simulink model "sfunction"  (R2022b)
settings: Solver=VariableStepAuto  StartTime=0.0  StopTime=2  RelTol=1e-3
libraries: fuzblock x2
settings Model: Creator=ericliu  LastModifiedBy=Lenovo
settings OptimizationCC: ReuseModelBlockBuffer=on
settings RTWCC: GPUComputeCapability=5.0

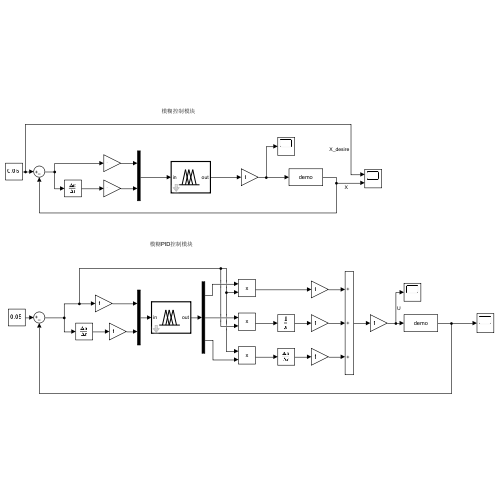
[thumbnail: Simulink's stored preview of the top-level diagram]
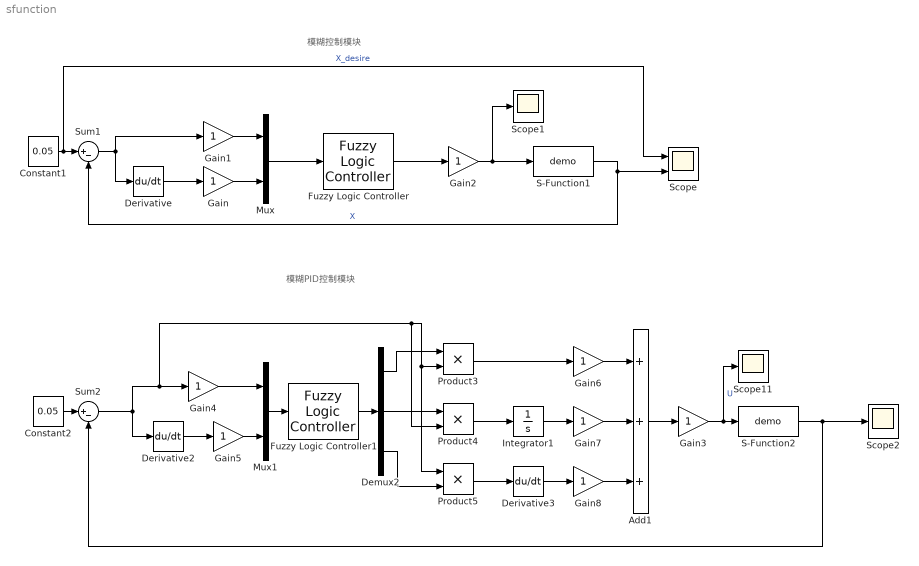
== system sfunction ==
  note: 模糊控制模块
  note: 模糊PID控制模块
  Add1 : Sum  Inputs=+++
  Constant1 : Constant  Value=0.05
  Constant2 : Constant  Value=0.05
  Demux2 : Demux  Outputs=3
  Derivative : Derivative
  Derivative2 : Derivative
  Derivative3 : Derivative
  Fuzzy Logic Controller : fuzblock/Fuzzy Logic  Controller  FIS='fuzzy1.fis'  OutputSampleNumber=101  DataType=double  FuzzifiedInputs=off  RuleFiringStrengths=off  RuleOutputs=off  AggregatedOutputs=off  SimulateUsing=Interpreted execution  OutOfRangeInputValueMessage=warning  NoRuleFiredMessage=warning  EmptyOutputFuzzySetMessage=warning
  Fuzzy Logic Controller1 : fuzblock/Fuzzy Logic  Controller  FIS='PIDfuzzy1.fis'  OutputSampleNumber=101  DataType=double  FuzzifiedInputs=off  RuleFiringStrengths=off  RuleOutputs=off  AggregatedOutputs=off  SimulateUsing=Interpreted execution  OutOfRangeInputValueMessage=warning  NoRuleFiredMessage=warning  EmptyOutputFuzzySetMessage=warning
  Gain{,1..8} (9 alike) : Gain
  Integrator1 : Integrator
  Mux : Mux  Inputs=2
  Mux1 : Mux  Inputs=2
  Product3 : Product
  Product4 : Product
  Product5 : Product
  S-Function1 : S-Function  FunctionName=demo  SFunctionDeploymentMode=off  EnableBusSupport=off
  S-Function2 : S-Function  FunctionName=demo  SFunctionDeploymentMode=off  EnableBusSupport=off
  Scope : Scope  NumInputPorts=2
  Scope1 : Scope
  Scope11 : Scope
  Scope2 : Scope
  Sum1 : Sum  Inputs=|+-
  Sum2 : Sum  Inputs=|+-
  wires:
  Mux/1 -> Fuzzy Logic Controller/1
  S-Function1/1 -> Scope/2, Sum1/2  "X"
  Sum1/1 -> Derivative/1, Gain1/1
  Gain1/1 -> Mux/1
  Derivative/1 -> Gain/1
  Gain/1 -> Mux/2
  Fuzzy Logic Controller/1 -> Gain2/1
  Gain2/1 -> Scope1/1, S-Function1/1
  Constant1/1 -> Scope/1, Sum1/1  "X_desire"
  Product4/1 -> Integrator1/1
  Fuzzy Logic Controller1/1 -> Demux2/1
  Gain4/1 -> Mux1/1
  Derivative2/1 -> Gain5/1
  Mux1/1 -> Fuzzy Logic Controller1/1
  Demux2/1 -> Product3/1
  Product5/1 -> Derivative3/1
  Add1/1 -> Gain3/1
  Integrator1/1 -> Gain7/1
  Gain8/1 -> Add1/3
  Product3/1 -> Gain6/1
  Gain7/1 -> Add1/2
  Derivative3/1 -> Gain8/1
  Gain3/1 -> Scope11/1, S-Function2/1  "U"
  Demux2/2 -> Product4/1
  Gain5/1 -> Mux1/2
  Demux2/3 -> Product5/2
  Gain6/1 -> Add1/1
  Sum2/1 -> Derivative2/1, Product5/1, Product3/2, Product4/2, Gain4/1
  Constant2/1 -> Sum2/1
  S-Function2/1 -> Scope2/1, Sum2/2
